simulink model "multiplexer4to1"  (R2025b)
settings: Solver=VariableStepAuto  StartTime=0.0  StopTime=10.0  RelTol=1e-3
settings Model: Creator=cyber  LastModifiedBy=cyber

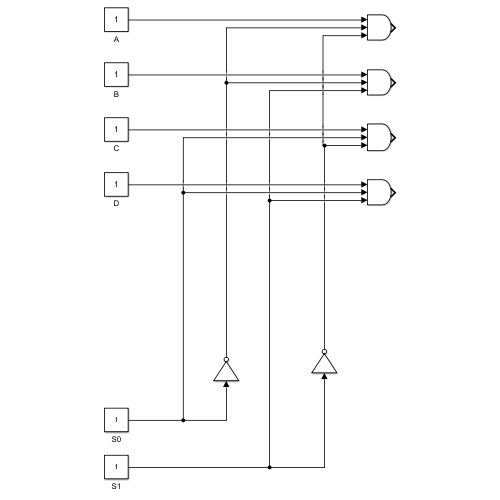
[thumbnail: Simulink's stored preview of the top-level diagram]
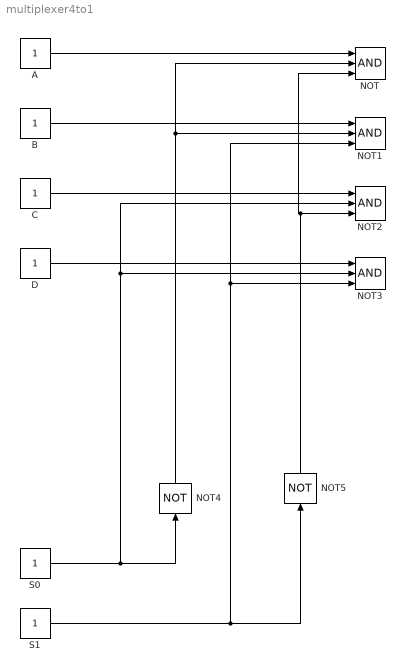
== system multiplexer4to1 ==
  A : Constant
  B : Constant
  C : Constant
  D : Constant
  NOT{,1..3} (4 alike) : Logic  Inputs=3  IconShape=distinctive  AllPortsSameDT=off  OutDataTypeStr=boolean
  NOT4 : Logic  Operator=NOT  IconShape=distinctive  AllPortsSameDT=off  OutDataTypeStr=boolean
  NOT5 : Logic  Operator=NOT  IconShape=distinctive  AllPortsSameDT=off  OutDataTypeStr=boolean
  S0 : Constant
  S1 : Constant
  wires:
  A/1 -> NOT/1
  S0/1 -> NOT4/1, NOT3/2, NOT2/2
  S1/1 -> NOT1/3, NOT3/3, NOT5/1
  B/1 -> NOT1/1
  NOT4/1 -> NOT/2, NOT1/2
  C/1 -> NOT2/1
  D/1 -> NOT3/1
  NOT5/1 -> NOT/3, NOT2/3
